simulink model "view_record_pci6221_20ms_COPY"  (R2015a)
settings: Solver=ode3  StartTime=0.0  StopTime=12  RelTol=1e-3
undefined symbols (not defined in the file or in its folder): National_Instruments, PCI
libraries: sldrtlib x2, simulink x1
settings Model: SimulationMode=external  CovHtmlReporting=off  ExtModeTrigDuration=100000  Creator=Alunos  LastModifiedBy=Alunos
settings HardwareCC: ProdBitPerPointer=64  ProdLargestAtomicFloat=Float  ProdIntDivRoundTo=Zero  ProdEndianess=LittleEndian  ProdHWDeviceType=Specified  TargetIntDivRoundTo=Zero  TargetEndianess=LittleEndian  TargetHWDeviceType=Intel->x86/Pentium
settings RTWCC: SystemTargetFile=rtwin.tlc  TemplateMakefile=rtwin.tmf  Description=Simulink Desktop Real-Time  RTWCompilerOptimization=on
settings CodeAppCC: MaxIdLength=95
settings RTWinTargetCC: TargetPreCompLibLocation=C:\Program Files\Polyspace\R2021a\toolbox\sldrt\lib\win64  ExtModeMexFile=sldrtext

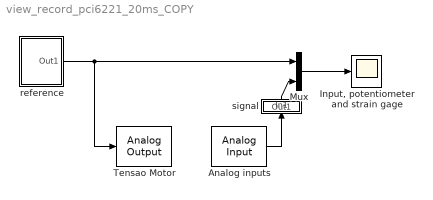
== system view_record_pci6221_20ms_COPY ==
  Analog inputs : sldrtlib/Analog Input  SampleTime=0.02  MaxMissedTicks=10  ShowMissedTicks=off  YieldWhenWaiting=off  DrvName=National_Instruments/PCI-6221  DrvAddress=4294967295  DrvOptions=[0 0 0 0 0]  Channels=1:4  RangeMode=1  VoltRange=1  DataType=1
      settings: AttributesFormatString=National Instruments\nPCI-6221 [auto]
  "Input, potentiometer and strain gage" : Scope
      settings: TickLabels=on  ShowLegends=on  YMin=-2.25  YMax=2  SampleInput=on  SampleTime=0.02
  Mux : Mux  Inputs=2
  Tensao Motor : sldrtlib/Analog Output  SampleTime=0.02  MaxMissedTicks=10  ShowMissedTicks=off  YieldWhenWaiting=off  DrvName=National_Instruments/PCI-6221  DrvAddress=4294967295  DrvOptions=[0 0 0 0 0]  Channels=1  RangeMode=1  VoltRange=1  InitialValue=0  FinalValue=0
      settings: AttributesFormatString=National Instruments\nPCI-6221 [auto]
  reference : Subsystem
  signal : Subsystem
  wires:
  Mux/1 -> "Input, potentiometer and strain gage"/1
  reference/1(Out1) -> Tensao Motor/1, Mux/1
  Analog inputs/1 -> signal/1(In1)
  signal/1(Out1) -> Mux/2

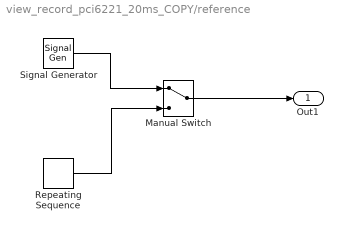
== system view_record_pci6221_20ms_COPY/reference ==
  Manual Switch : ManualSwitch
  Repeating Sequence : simulink/Sources/Repeating Sequence  rep_seq_t=[0 0.9999 1 1.9999 2 2.9999 3 4]  rep_seq_y=[1 1 0 0 -1 -1 0 0]
  Signal Generator : SignalGenerator  WaveForm=square  Frequency=0.5
  Out1 : Outport
  wires:
  Signal Generator/1 -> Manual Switch/1
  Repeating Sequence/1 -> Manual Switch/2
  Manual Switch/1 -> Out1/1

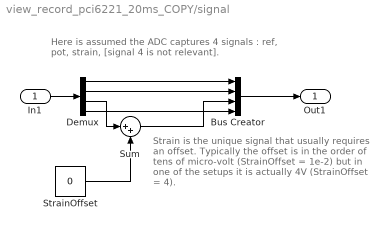
== system view_record_pci6221_20ms_COPY/signal ==
  note: Strain is the unique signal that usually requires an offset. Typically the offset is in the order of tens of micro-volt (StrainOffset = 1e-2) but in one of the setups it is actually 4V (StrainOffset = 4).
  note: Here is assumed the ADC captures 4 signals :
      | ref, pot, strain, [signal 4 is not relevant].
  In1 : Inport
  Bus Creator : BusCreator
  Demux : Demux
  StrainOffset : Constant  Value=0
  Sum : Sum  Inputs=|++
  Out1 : Outport
  wires:
  In1/1 -> Demux/1
  Bus Creator/1 -> Out1/1
  Demux/1 -> Bus Creator/1
  Demux/2 -> Bus Creator/2
  Demux/4 -> Bus Creator/4
  Demux/3 -> Sum/1
  Sum/1 -> Bus Creator/3
  StrainOffset/1 -> Sum/2
